simulink model "LyRStateCtrl"  (R2018b)
settings: Solver=FixedStepDiscrete  StartTime=0.0  StopTime=10.0  FixedStep=0.01  RelTol=1e-3
libraries: StateCtrlLib x1
settings Model: Creator=sn2xws  LastModifiedBy=sn2xws
settings DataIOCC: SaveFormat=StructureWithTime
settings OptimizationCC: DefaultParameterBehavior=Inlined  EnhancedBackFolding=on  PassReuseOutputArgsAs=Individual arguments  ZeroExternalMemoryAtStartup=off  ZeroInternalMemoryAtStartup=off  OptimizeBlockOrder=speed  DifferentSizesBufferReuse=on  OptimizationCustomize=off
settings DebuggingCC: ParameterTunabilityLossMsg=error
settings ModelReferenceCC: ModelReferenceNumInstancesAllowed=Single
settings SFSimCC: MATLABDynamicMemAlloc=off
settings RTWCC: SystemTargetFile=autosar.tlc  GenCodeOnly=on  TemplateMakefile=ert_default_tmf  Description=AUTOSAR  GenerateReport=on  IncludeHyperlinkInReport=on  LaunchReport=on  GenerateTraceInfo=on  GenerateTraceReport=on  GenerateTraceReportSl=on  GenerateTraceReportSf=on  GenerateTraceReportEml=on
settings CodeAppCC: ForceParamTrailComments=on  IgnoreCustomStorageClasses=off  OperatorAnnotations=on  SimulinkDataObjDesc=on  SFDataObjDesc=on  InsertBlockDesc=on
settings STFCustomTargetCC: TargetLangStandard=C99 (ISO)  MultiwordLength=256  ParMdlRefBuildCompliant=on  CompOptLevelCompliant=on  IncludeMdlTerminateFcn=off  CombineOutputUpdateFcns=on  SuppressErrorStatus=on  ERTCustomFileBanners=on  SupportNonFinite=off  SupportComplex=off  SupportContinuousTime=off  SupportNonInlinedSFcns=off  RemoveResetFunc=on  MATLABClassNameForMDSCustomization=Simulink.SoftwareTarget.ERTCustomization  AutosarCompliant=on  UseToolchainInfoCompliant=on  LookupTableObjectStructAxisOrder=2,1,3,4,...  LUTObjectStructOrderEvenSpacing=Size,Table,Breakpoints  SystemTargetFile=autosar.tlc
settings ERTTargetCC: TargetLangStandard=C99 (ISO)  ConcurrentExecutionCompliant=off  IncludeMdlTerminateFcn=off  SuppressErrorStatus=on  SupportNonFinite=off  SupportComplex=off  ModelStepFunctionPrototypeControlCompliant=off  CPPClassGenCompliant=off  AutosarCompliant=on  LookupTableObjectStructAxisOrder=2,1,3,4,...  LUTObjectStructOrderEvenSpacing=Size,Table,Breakpoints  InlinedParameterPlacement=NonHierarchical  ERTCustomFileTemplate=example_file_process.tlc

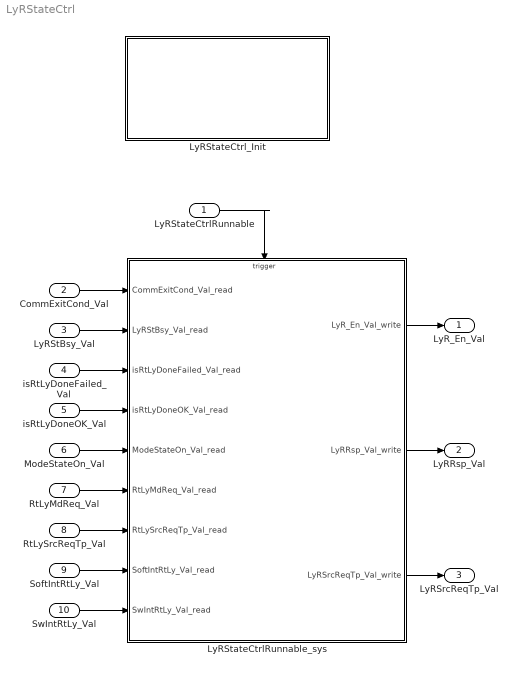
== system LyRStateCtrl ==
  LyRStateCtrlRunnable : Inport  SampleTime=0.01  OutputFunctionCall=on
  CommExitCond_Val : Inport  Port=2  OutDataTypeStr=boolean  PortDimensions=1
  LyRStBsy_Val : Inport  Port=3  OutDataTypeStr=boolean  PortDimensions=1
  isRtLyDoneFailed_Val : Inport  Port=4  OutDataTypeStr=boolean  PortDimensions=1
  isRtLyDoneOK_Val : Inport  Port=5  OutDataTypeStr=boolean  PortDimensions=1
  ModeStateOn_Val : Inport  Port=6  OutDataTypeStr=boolean  PortDimensions=1
  RtLyMdReq_Val : Inport  Port=7  OutDataTypeStr=boolean  PortDimensions=1
  RtLySrcReqTp_Val : Inport  Port=8  OutDataTypeStr=Enum: SrcReqTp1  PortDimensions=1
  SoftIntRtLy_Val : Inport  Port=9  OutDataTypeStr=IntEnable  PortDimensions=1
  SwIntRtLy_Val : Inport  Port=10  OutDataTypeStr=IntEnable  PortDimensions=1
  LyRStateCtrlRunnable_sys : Subsystem
  LyRStateCtrl_Init : Subsystem
  LyR_En_Val : Outport  OutDataTypeStr=boolean  PortDimensions=1
  LyRRsp_Val : Outport  Port=2  OutDataTypeStr=Enum: MdRspLocal1  PortDimensions=1
  LyRSrcReqTp_Val : Outport  Port=3  OutDataTypeStr=Enum: SrcReqTp1  PortDimensions=1
  wires:
  CommExitCond_Val/1 -> LyRStateCtrlRunnable_sys/1(CommExitCond_Val_read)
  LyRStBsy_Val/1 -> LyRStateCtrlRunnable_sys/2(LyRStBsy_Val_read)
  isRtLyDoneFailed_Val/1 -> LyRStateCtrlRunnable_sys/3(isRtLyDoneFailed_Val_read)
  isRtLyDoneOK_Val/1 -> LyRStateCtrlRunnable_sys/4(isRtLyDoneOK_Val_read)
  ModeStateOn_Val/1 -> LyRStateCtrlRunnable_sys/5(ModeStateOn_Val_read)
  RtLyMdReq_Val/1 -> LyRStateCtrlRunnable_sys/6(RtLyMdReq_Val_read)
  RtLySrcReqTp_Val/1 -> LyRStateCtrlRunnable_sys/7(RtLySrcReqTp_Val_read)
  SoftIntRtLy_Val/1 -> LyRStateCtrlRunnable_sys/8(SoftIntRtLy_Val_read)
  SwIntRtLy_Val/1 -> LyRStateCtrlRunnable_sys/9(SwIntRtLy_Val_read)
  LyRStateCtrlRunnable_sys/1(LyR_En_Val_write) -> LyR_En_Val/1
  LyRStateCtrlRunnable_sys/2(LyRRsp_Val_write) -> LyRRsp_Val/1
  LyRStateCtrlRunnable_sys/3(LyRSrcReqTp_Val_write) -> LyRSrcReqTp_Val/1
  LyRStateCtrlRunnable/1 -> LyRStateCtrlRunnable_sys/Trigger

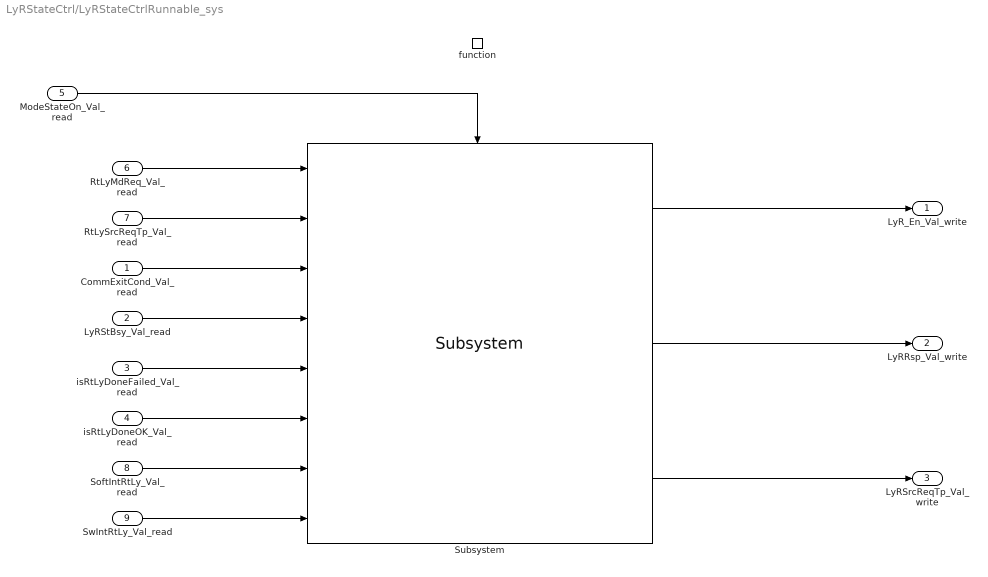
== system LyRStateCtrl/LyRStateCtrlRunnable_sys ==
  CommExitCond_Val_read : Inport
  LyRStBsy_Val_read : Inport  Port=2
  isRtLyDoneFailed_Val_read : Inport  Port=3
  isRtLyDoneOK_Val_read : Inport  Port=4
  ModeStateOn_Val_read : Inport  Port=5
  RtLyMdReq_Val_read : Inport  Port=6
  RtLySrcReqTp_Val_read : Inport  Port=7
  SoftIntRtLy_Val_read : Inport  Port=8  OutDataTypeStr=IntEnable
  SwIntRtLy_Val_read : Inport  Port=9  OutDataTypeStr=IntEnable
  function : TriggerPort  TriggerType=function-call  VariantControl=(inherit)  SampleTimeType=periodic  SampleTime=-1
  Subsystem : StateCtrlLib/Subsystem  SystemSampleTime=-1
  LyR_En_Val_write : Outport
      settings: EnsureOutportIsVirtual=on
  LyRRsp_Val_write : Outport  Port=2
      settings: EnsureOutportIsVirtual=on
  LyRSrcReqTp_Val_write : Outport  Port=3
      settings: EnsureOutportIsVirtual=on
  wires:
  Subsystem/2 -> LyRRsp_Val_write/1
  Subsystem/1 -> LyR_En_Val_write/1
  Subsystem/3 -> LyRSrcReqTp_Val_write/1
  RtLyMdReq_Val_read/1 -> Subsystem/1
  RtLySrcReqTp_Val_read/1 -> Subsystem/2
  SoftIntRtLy_Val_read/1 -> Subsystem/7
  CommExitCond_Val_read/1 -> Subsystem/3
  LyRStBsy_Val_read/1 -> Subsystem/4
  SwIntRtLy_Val_read/1 -> Subsystem/8
  isRtLyDoneFailed_Val_read/1 -> Subsystem/5
  isRtLyDoneOK_Val_read/1 -> Subsystem/6
  ModeStateOn_Val_read/1 -> Subsystem/Enable

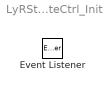
== system LyRStateCtrl/LyRStateCtrl_Init ==
  Event Listener : EventListener  EventName=reset
